simulink model "Multi_agent_system"  (R2016b)
settings: Solver=VariableStepAuto  StartTime=0.0  StopTime=10  RelTol=1e-3
undefined symbols (not defined in the file or in its folder): A1, n, r, x_initial
settings Model: Creator=kvlton  LastModifiedBy=kvlton

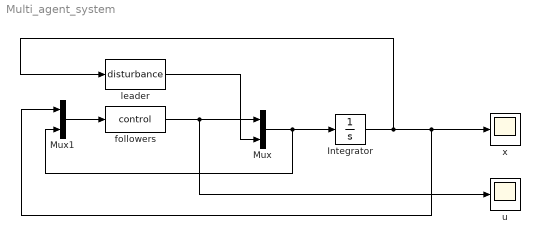
== system Multi_agent_system ==
  Integrator : Integrator  InitialCondition=x_initial
  Mux : Mux  Inputs=2
  Mux1 : Mux  Inputs=2
  followers : S-Function  FunctionName=control  Parameters=A1,A1,n,r  SFunctionDeploymentMode=off  EnableBusSupport=off
  leader : S-Function  FunctionName=disturbance  Parameters=n  SFunctionDeploymentMode=off  EnableBusSupport=off
  u : Scope
  x : Scope
  wires:
  Integrator/1 -> leader/1, Mux1/1, x/1
  Mux/1 -> Integrator/1, Mux1/2
  followers/1 -> Mux/1, u/1
  Mux1/1 -> followers/1
  leader/1 -> Mux/2
